simulink model "FWMAV_DirectDrive"  (R2022b)
settings: Solver=ode4  StartTime=0.0  StopTime=t_stop  FixedStep=dt  RelTol=1e-3
values from neighbouring files (symbols this model uses):
  bm = 3.6e-6    (= 3.6e-06)    [FWMAV_Parameters.m]
  J_total = Jm + Jw    (= 4.44435202442e-07)    [FWMAV_Parameters.m]    (also in Motor_Selection_fmincon.m = motor.Jm + Jw; Optimize_DirectDrive.m = Jm + Jw; old_fmincon.m = motor.Jm + Jw)
  Kb = 0.01    [FWMAV_Parameters.m]
  KDD = J_total * (2*pi*freq)^2    (= 0.0100138362891)    [FWMAV_Parameters.m]    (also in Motor_Selection_fmincon.m = J_total * (2*pi*freq)^2; Optimize_DirectDrive.m = J_total * (2*pi*freq)^2; old_fmincon.m = J_total * (2*pi*freq)^2)
  Kt = 0.01    [FWMAV_Parameters.m]
  La = 0.029    [FWMAV_Parameters.m]
  omega = 2*pi*freq    (= 150.105296989)    [FWMAV_Parameters.m]
  Ra = 9    [FWMAV_Parameters.m]
  V_amplitude = 5    [FWMAV_Parameters.m]    (also in Motor_Selection_fmincon.m; Optimize_DirectDrive.m; old_fmincon.m = 3)
settings Model: Creator=Saatvik  LastModifiedBy=Saatvik

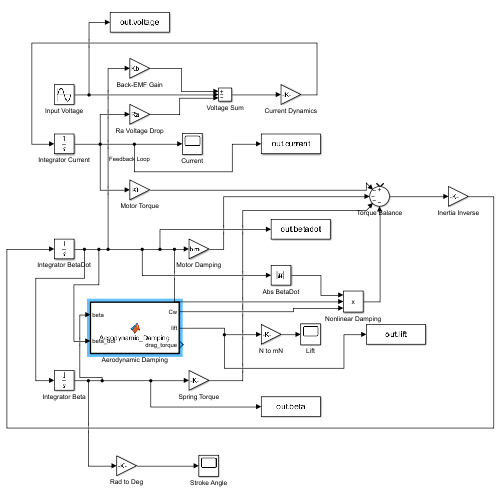
[thumbnail: Simulink's stored preview of the top-level diagram]
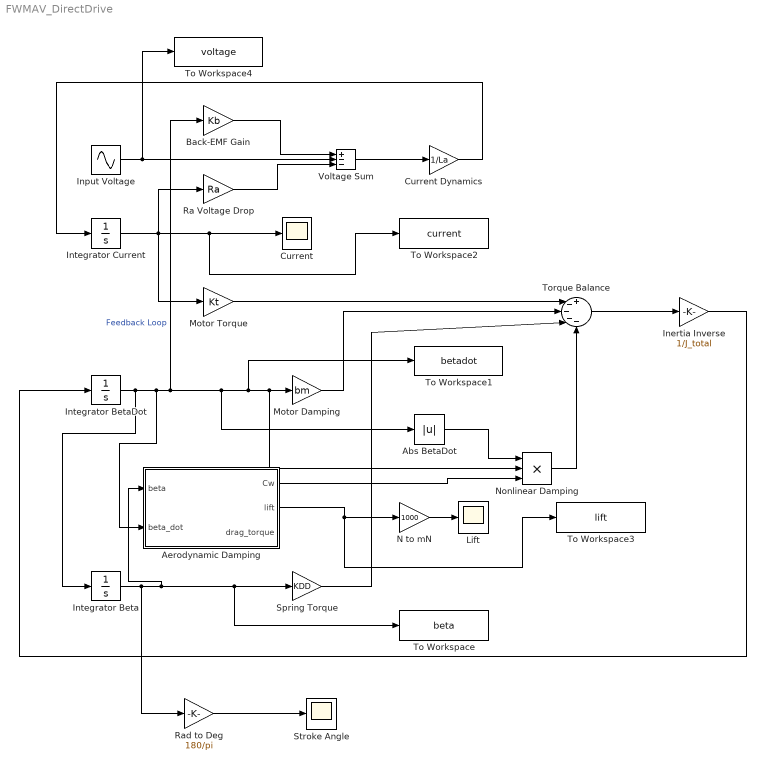
== system FWMAV_DirectDrive ==
  Abs BetaDot : Abs  SaturateOnIntegerOverflow=off
  Aerodynamic Damping : MATLAB Function  TreatAsAtomicUnit=on
  Back-EMF Gain : Gain  Gain=Kb
  Current : Scope
  Current Dynamics : Gain  Gain=1/La
  Inertia Inverse : Gain  Gain=1/J_total
  Input Voltage : Sin  Amplitude=V_amplitude  Frequency=omega  SampleTime=0
  Integrator Beta : Integrator
  Integrator BetaDot : Integrator
  Integrator Current : Integrator
  Lift : Scope
  Motor Damping : Gain  Gain=bm
  Motor Torque : Gain  Gain=Kt
  N to mN : Gain  Gain=1000
  Nonlinear Damping : Product  Inputs=3
  Ra Voltage Drop : Gain  Gain=Ra
  Rad to Deg : Gain  Gain=180/pi
  Spring Torque : Gain  Gain=KDD
  Stroke Angle : Scope
  To Workspace : ToWorkspace  VariableName=beta  SaveFormat=Structure With Time  SampleTime=-1
  To Workspace1 : ToWorkspace  VariableName=betadot  SaveFormat=Structure With Time  SampleTime=-1
  To Workspace2 : ToWorkspace  VariableName=current  SaveFormat=Structure With Time  SampleTime=-1
  To Workspace3 : ToWorkspace  VariableName=lift  SaveFormat=Structure With Time  SampleTime=-1
  To Workspace4 : ToWorkspace  VariableName=voltage  SaveFormat=Structure With Time  SampleTime=-1
  Torque Balance : Sum  Inputs=+----
  Voltage Sum : Sum  Inputs=+--
  wires:
  Input Voltage/1 -> To Workspace4/1, Voltage Sum/2
  Ra Voltage Drop/1 -> Voltage Sum/3
  Back-EMF Gain/1 -> Voltage Sum/1
  Voltage Sum/1 -> Current Dynamics/1
  Current Dynamics/1 -> Integrator Current/1
  Integrator Current/1 -> To Workspace2/1, Current/1, Motor Torque/1, Ra Voltage Drop/1
  Motor Torque/1 -> Torque Balance/2
  Integrator BetaDot/1 -> Integrator Beta/1, Aerodynamic Damping/2(beta_dot), Back-EMF Gain/1, Abs BetaDot/1, To Workspace1/1, Nonlinear Damping/2, Motor Damping/1  "Feedback Loop"
  Motor Damping/1 -> Torque Balance/3
  Integrator Beta/1 -> Rad to Deg/1, Aerodynamic Damping/1(beta), To Workspace/1, Spring Torque/1
  Spring Torque/1 -> Torque Balance/4
  Aerodynamic Damping/1(Cw) -> Nonlinear Damping/3
  Abs BetaDot/1 -> Nonlinear Damping/1
  Nonlinear Damping/1 -> Torque Balance/5
  Torque Balance/1 -> Inertia Inverse/1
  Inertia Inverse/1 -> Integrator BetaDot/1
  Aerodynamic Damping/2(lift) -> To Workspace3/1, N to mN/1
  Rad to Deg/1 -> Stroke Angle/1
  N to mN/1 -> Lift/1

== matlab function FWMAV_DirectDrive/Aerodynamic Damping ==
  data: beta input; Cw output; beta_dot input; lift output; drag_torque output
function [Cw, lift, drag_torque] = Aerodynamic_Damping(beta, beta_dot)
    % Parameters
    Calpha = 5e-3;
    rho = 1.225;
    Le = 0.06846;
    Lc = Le / 3;
    Lb = 0.010;
    
    % Angle of attack (Eq. 10)
    alpha = pi/2 - Calpha * abs(beta_dot);
    alpha = max(alpha, pi/4);
    
    % Lift and drag coefficients (Eqs. 8, 9)
    CL = 0.225 + 1.58 * sin(2.13*alpha - 0.1257);
    CD = 1.92 - 1.55 * cos(2.04*alpha - 0.1714);
    
    % Blade element integration
    n_elements = 100;
    r = linspace(Lb/2, Le + Lb/2, n_elements);
    dr = r(2) - r(1);
    
    lift_total = 0;
    drag_torque_total = 0;  % Changed name
    Cw_sum = 0;
    
    for i = 1:n_elements
        c_r = Lc * sqrt(max(0, 1 - ((r(i) - Lb/2) / Le)^2));
        Ar = c_r * dr;
        Vr = abs(r(i) * beta_dot);
        
        Lr = 0.5 * rho * Vr^2 * Ar * CL;
        Dr = 0.5 * rho * Vr * abs(Vr) * Ar * CD;
        
        lift_total = lift_total + Lr;
        drag_torque_total = drag_torque_total + Dr * r(i);  % MULTIPLY by r(i)
        
        Cw_sum = Cw_sum + 0.5 * rho * r(i)^3 * Ar;
    end
    
    Cw = CD * Cw_sum;
    lift = lift_total;
    drag_torque = drag_torque_total;  % This is now torque [Nm]
end
